simulink model "models"  (R2016a)
settings: Solver=VariableStepAuto  StartTime=0.0  StopTime=10.0  RelTol=1e-3
settings Model: Creator=Ravel  LastModifiedBy=Ravel

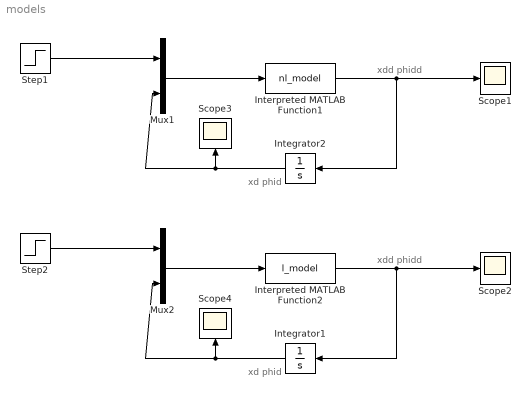
== system models ==
  note: xd phid
  note: xdd phidd
  note: xd phid
  note: xdd phidd
  Integrator1 : Integrator  InitialCondition=[1;2;3;3]
  Integrator2 : Integrator  InitialCondition=[1;2;3;3]
  Interpreted MATLAB Function1 : MATLABFcn  MATLABFcn=nl_model
  Interpreted MATLAB Function2 : MATLABFcn  MATLABFcn=l_model
  Mux1 : Mux  Inputs=2
  Mux2 : Mux  Inputs=2
  Scope{1..4} (4 alike) : Scope
  Step1 : Step  Time=0  After=0  SampleTime=0  ZeroCross=off
  Step2 : Step  Time=0  After=0  SampleTime=0  ZeroCross=off
  wires:
  Mux1/1 -> Interpreted MATLAB Function1/1
  Interpreted MATLAB Function1/1 -> Integrator2/1, Scope1/1
  Integrator2/1 -> Mux1/2, Scope3/1
  Step1/1 -> Mux1/1
  Mux2/1 -> Interpreted MATLAB Function2/1
  Interpreted MATLAB Function2/1 -> Scope2/1, Integrator1/1
  Integrator1/1 -> Scope4/1, Mux2/2
  Step2/1 -> Mux2/1
